simulink model "PV_MPPT_DesktopSim_ST"  (R2018b)
settings: Solver=ode23tb  StartTime=0.0  StopTime=inf  MaxStep=1e-4  RelTol=1e-3
PreLoadFcn:
  | load('EmulatedPV_LowPowerData.mat');
  | 
  | numIrr = 10;
  | ArrayPower = ArrayCurrent.*ArrayVoltage;
InitFcn:
  | Ts = 1e-4;
  | Tc = Ts;
undefined symbols (not defined in the file): ArrayCurrent, ArrayVoltage, DiscIntNeverNeededParam, Irradiance, Tdata
libraries: powerlib x18, simulink x3, powerlib_meascontrol x3
settings Model: Creator=mmishra  LastModifiedBy=jlesage
settings DebuggingCC: LibraryContextMissingDiagnostic=none
settings SFSimCC: SimUseLocalCustomCode=off
settings RTWCC: RTWUseLocalCustomCode=off

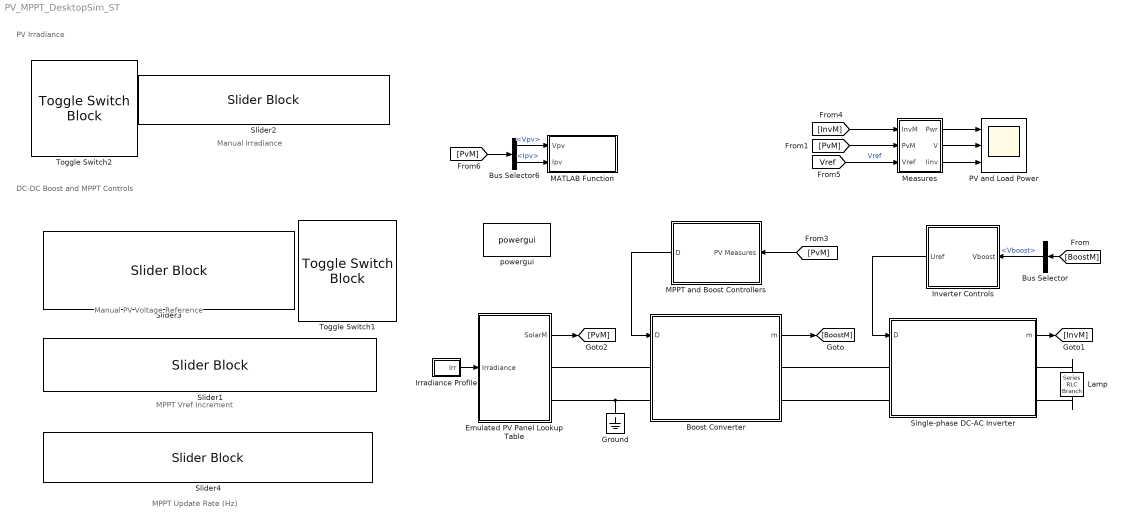
== system PV_MPPT_DesktopSim_ST ==
  note: Manual Irradiance
  note: PV Irradiance
  note: MPPT Update Rate (Hz)
  note: MPPT Vref Increment
  note: DC-DC Boost and MPPT Controls
  note: Manual PV Voltage Reference
  Boost Converter : Subsystem
  Bus Selector : BusSelector  OutputSignals=Vboost
  Bus Selector6 : BusSelector  OutputSignals=Vpv,Ipv
  Emulated PV Panel Lookup Table : Subsystem
      mask Display:
      | image(imread('panel.jpg'))
      | color('yellow')
      | port_label('input',1,'Ir')
      | port_label('output',1,'m')
      | port_label('Rconn',1,'A')
      | port_label('Rconn',2,'B')
  Ground : powerlib/Elements/Ground  LConnTagsString=a
      settings: SourceProductName=Simscape Electrical
  Inverter Controls : Subsystem
  Irradiance Profile : Subsystem
  Lamp : powerlib/Elements/Series RLC Branch  LConnTagsString=__new0  RConnTagsString=__new0  BranchType=R  Resistance=11.5  Inductance=1e-3  SetiL0=off  InitialCurrent=0  Capacitance=1e-6  Setx0=off  InitialVoltage=0  Measurements=None
      settings: SourceProductName=Simscape Electrical
  MATLAB Function : MATLAB Function  TreatAsAtomicUnit=on  SystemSampleTime=1/20
  MPPT and Boost Controllers : Subsystem
  Measures : Subsystem
  PV and Load Power : Scope  NumInputPorts=3
  Single-phase DC-AC Inverter : Subsystem
  Slider1 : SliderBlock  WebBlockId=613  ScaleMax=0.5  TickInterval=0.10000000000000001
  Slider2 : SliderBlock  WebBlockId=612  ScaleMax=0.5  TickInterval=0.10000000000000001
  Slider3 : SliderBlock  WebBlockId=614  ScaleMin=1  ScaleMax=10  TickInterval=1
  Slider4 : SliderBlock  WebBlockId=615  ScaleMin=25  ScaleMax=250  TickInterval=25
  Toggle Switch1 : ToggleSwitchBlock  WebBlockId=610  LabelPosition=Hide
      settings: Values={{'Manual Vref', 'Enable MPPT'}, [0 1]}
  Toggle Switch2 : ToggleSwitchBlock  WebBlockId=611  LabelPosition=Hide
      settings: Values={{'Use Profile', 'Set Irradiance'}, [0 1]}
  powergui : powerlib/powergui  Priority=1  SimulationMode=Discrete  SampleTime=Ts  frequency=60  Iterations=50  frequencyindice=0  Pbase=100e6  ErrMax=1e-4  UnitsV=kV  UnitsW=MW  buscounter=0  FunctionMessages=off  echomessages=off  EnableUseOfTLC=off  CurrentSourceSwitches=off  DisableSnubberDevices=off  DisableRonSwitches=off  DisableVfSwitches=off  DisplayEquations=off  SolverType=Tustin/Backward Euler (TBE)  Interpol=off  ExternalGateDelay=off  methode=off  Ts=100  x0status=blocks  SPID=on  SwTol=0  HookPort=off  RestoreLinks=warning  ResistiveCurrentMeasurement=off  Frange=[0:2:500]  Ylog=off  Xlog=on  ShowGrid=off  save=off  variable=ZData  structure=0  ZoomFFT=off  StartTime=0.0  cycles=1  DisplayStyle=1  fundamental=60  FreqAxis=off  MaxFrequency=1000  frequencyindicesteady=1  RmsSteady=1  display=off
      settings: SourceProductName=Simscape Electrical
  wires:
  Irradiance Profile/1(Irr) -> Emulated PV Panel Lookup Table/1(Irradiance)
  Single-phase DC-AC Inverter/1(m) -> [InvM]
  Emulated PV Panel Lookup Table/1(SolarM) -> [PvM]
  MPPT and Boost Controllers/1(D) -> Boost Converter/1(D)
  Boost Converter/1(m) -> [BoostM]
  [PvM] -> MPPT and Boost Controllers/1(PV Measures)
  Bus Selector/1 -> Inverter Controls/1(Vboost)  "<Vboost>"
  Inverter Controls/1(Uref) -> Single-phase DC-AC Inverter/1(D)
  [BoostM] -> Bus Selector/1
  Bus Selector6/1 -> MATLAB Function/1(Vpv)  "<Vpv>"
  Bus Selector6/2 -> MATLAB Function/2(Ipv)  "<Ipv>"
  [PvM] -> Bus Selector6/1
  [InvM] -> Measures/1(InvM)
  [PvM] -> Measures/2(PvM)
  [Vref] -> Measures/3(Vref)  "Vref"
  Measures/1(Pwr) -> PV and Load Power/1
  Measures/2(V) -> PV and Load Power/2
  Measures/3(Iinv) -> PV and Load Power/3
  connections:
  Ground/LConn1 -- Emulated PV Panel Lookup Table/RConn2 -- Boost Converter/LConn2
  Emulated PV Panel Lookup Table/RConn1 -- Boost Converter/LConn1
  Lamp/RConn1 -- Single-phase DC-AC Inverter/RConn2
  Single-phase DC-AC Inverter/LConn1 -- Boost Converter/RConn1
  Single-phase DC-AC Inverter/LConn2 -- Boost Converter/RConn2
  Lamp/LConn1 -- Single-phase DC-AC Inverter/RConn1

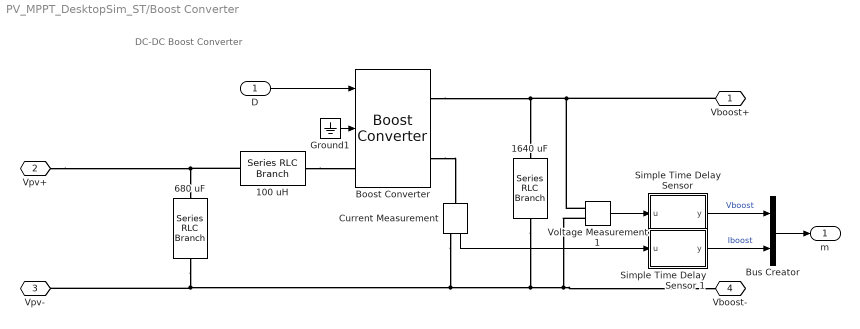
== system PV_MPPT_DesktopSim_ST/Boost Converter ==
  note: DC-DC Boost Converter
  D : Inport
  100 uH : powerlib/Elements/Series RLC Branch  LConnTagsString=__new0  RConnTagsString=__new0  BranchType=L  Resistance=1  Inductance=100e-6  SetiL0=off  InitialCurrent=0  Capacitance=1e-6  Setx0=off  InitialVoltage=0  Measurements=None
      settings: SourceProductName=Simscape Electrical
  1640 uF : powerlib/Elements/Series RLC Branch  LConnTagsString=__new0  RConnTagsString=__new0  BranchType=C  Resistance=1  Inductance=1e-3  SetiL0=off  InitialCurrent=0  Capacitance=1640e-6  Setx0=off  InitialVoltage=30  Measurements=None
      settings: SourceProductName=Simscape Electrical
  680 uF : powerlib/Elements/Series RLC Branch  LConnTagsString=__new0  RConnTagsString=__new0  BranchType=C  Resistance=1e-3  Inductance=1e-3  SetiL0=off  InitialCurrent=0  Capacitance=680e-6  Setx0=off  InitialVoltage=20  Measurements=None
      settings: SourceProductName=Simscape Electrical
  "Boost Converter " : powerlib/Power Electronics/Boost Converter  ModelType=Average model (D-controlled)  Ron=1e-3  Rs=1e6  Cs=inf  Vforward=[0,0.8]  Ron_Diode=1e-3  Rs_Diode=1e6  Cs_Diode=inf  Vf_Diode=0.8  Rs_CurrentSource=inf
      settings: SourceProductName=Simscape Electrical  SourceProductBaseCode=PS
  Bus Creator : BusCreator  Inputs=2
  Current Measurement : powerlib/Measurements/Current Measurement  PhasorSimulation=off  OutputType=Complex  PSBequivalent=0
      settings: SourceProductName=Simscape Electrical
  Ground1 : Ground
  "Simple Time Delay Sensor " : Subsystem  mask{Ts=Ts, Tau=0.0001}
      mask prompts: Ts "Sample Time, [s]"; Tau "Time Constant, Tau [s]"
      mask help: Simple Sensor
      mask Display: fprintf('1\n------------\n(1 + s Tau)');
  Simple Time Delay Sensor 1 : Subsystem  mask{Ts=Ts, Tau=0.0001}
      mask prompts: Ts "Sample Time, [s]"; Tau "Time Constant, Tau [s]"
      mask help: Simple Sensor
      mask Display: fprintf('1\n------------\n(1 + s Tau)');
  Voltage Measurement1 : powerlib/Measurements/Voltage Measurement  PhasorSimulation=off  OutputType=Complex  PSBequivalent=0
      settings: SourceProductName=Simscape Electrical
  Vboost+ : PMIOPort  Side=Right
  Vpv+ : PMIOPort  Port=2  Side=Left
  Vpv- : PMIOPort  Port=3  Side=Left
  Vboost- : PMIOPort  Port=4  Side=Right
  m : Outport
  wires:
  Ground1/1 -> "Boost Converter "/2
  Current Measurement/1 -> Simple Time Delay Sensor 1/1(u)
  Voltage Measurement1/1 -> "Simple Time Delay Sensor "/1(u)
  Bus Creator/1 -> m/1
  "Simple Time Delay Sensor "/1(y) -> Bus Creator/1  "Vboost"
  Simple Time Delay Sensor 1/1(y) -> Bus Creator/2  "Iboost"
  D/1 -> "Boost Converter "/1
  connections:
  100 uH/LConn1 -- Vpv+/RConn1 -- 680 uF/LConn1
  "Boost Converter "/RConn2 -- Current Measurement/LConn1
  100 uH/RConn1 -- "Boost Converter "/LConn1
  Voltage Measurement1/LConn1 -- Vboost+/RConn1 -- "Boost Converter "/RConn1 -- 1640 uF/LConn1
  680 uF/RConn1 -- Vboost-/RConn1 -- Voltage Measurement1/LConn2 -- 1640 uF/RConn1 -- Current Measurement/RConn1 -- Vpv-/RConn1

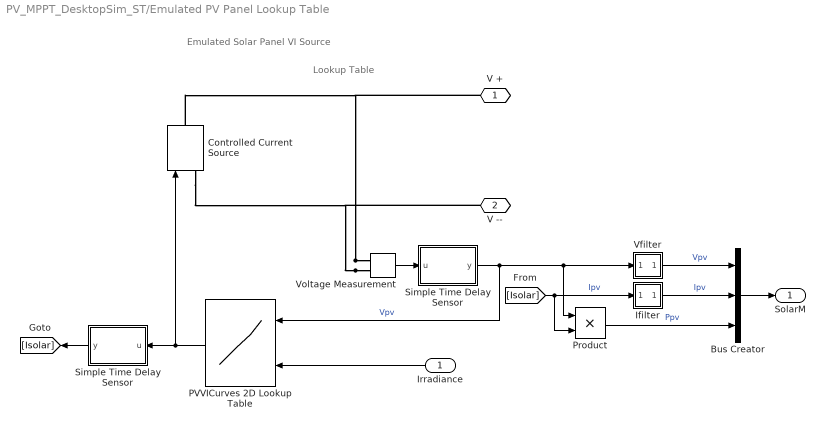
== system PV_MPPT_DesktopSim_ST/Emulated PV Panel Lookup Table ==
  note: Lookup Table
  note: Emulated Solar Panel VI Source
  Irradiance : Inport
  Bus Creator : BusCreator  Inputs=3
  Controlled Current Source : powerlib/Electrical Sources/Controlled Current Source  Initialize=on  Source_Type=AC  Amplitude=0  Phase=0  Frequency=0  Measurements=None
      settings: SourceProductName=Simscape Electrical
  Ifilter : Subsystem  mask{Tf=0.01}
      mask prompts: Tf "Filter Time Constant"
  PVVICurves 2D Lookup Table : Lookup_n-D  BreakpointsForDimension1=ArrayVoltage  BreakpointsForDimension2=Irradiance  Table=ArrayCurrent  InternalRulePriority=Speed  RndMeth=Simplest  InputSameDT=on
  Product : Product
  Simple Time Delay Sensor : Subsystem  mask{Ts=Ts, Tau=0.0001}
      mask prompts: Ts "Sample Time, [s]"; Tau "Time Constant, Tau [s]"
      mask help: Simple Sensor
      mask Display: fprintf('1\n------------\n(1 + s Tau)');
  "Simple Time Delay Sensor " : Subsystem  mask{Ts=Ts, Tau=0.0001}
      mask prompts: Ts "Sample Time, [s]"; Tau "Time Constant, Tau [s]"
      mask help: Simple Sensor
      mask Display: fprintf('1\n------------\n(1 + s Tau)');
  Vfilter : Subsystem  mask{Tf=0.01}
      mask prompts: Tf "Filter Time Constant"
  Voltage Measurement : powerlib/Measurements/Voltage Measurement  PhasorSimulation=off  OutputType=Complex  PSBequivalent=0
      settings: SourceProductName=Simscape Electrical
  V + : PMIOPort  Side=Right
  V -- : PMIOPort  Port=2  Side=Right
  SolarM : Outport
  wires:
  Irradiance/1 -> PVVICurves 2D Lookup Table/2
  PVVICurves 2D Lookup Table/1 -> Simple Time Delay Sensor/1(u), Controlled Current Source/1
  Bus Creator/1 -> SolarM/1
  [Isolar] -> Product/2, Ifilter/1(u)  "Ipv"
  Product/1 -> Bus Creator/3  "Ppv"
  Simple Time Delay Sensor/1(y) -> [Isolar]
  "Simple Time Delay Sensor "/1(y) -> Product/1, Vfilter/1(u), PVVICurves 2D Lookup Table/1  "Vpv"
  Voltage Measurement/1 -> "Simple Time Delay Sensor "/1(u)
  Vfilter/1(y) -> Bus Creator/1  "Vpv"
  Ifilter/1(y) -> Bus Creator/2  "Ipv"
  connections:
  Voltage Measurement/LConn2 -- Controlled Current Source/LConn1 -- V --/RConn1
  Voltage Measurement/LConn1 -- Controlled Current Source/RConn1 -- V +/RConn1

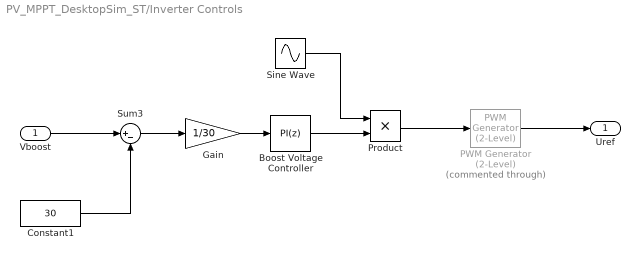
== system PV_MPPT_DesktopSim_ST/Inverter Controls ==
  Vboost : Inport
  Boost Voltage Controller : simulink/Continuous/PID Controller  Controller=PI  Form=Parallel  TimeDomain=Discrete-time  SampleTime=Tc  IntegratorMethod=Forward Euler  FilterMethod=Forward Euler  ControllerParametersSource=internal  P=3  I=250  D=0  UseFilter=on  N=100  TunerSelectOption=Transfer Function Based (PID Tuner App)  InitialConditionSource=internal  InitialConditionForIntegrator=1  InitialConditionForFilter=0  DifferentiatorICPrevScaledInput=0  ExternalReset=none  TrackingMode=off  Kt=1  LimitOutput=on  UpperSaturationLimit=1  LowerSaturationLimit=0  LinearizeAsGain=on  AntiWindupMode=clamping  Kb=1  POutMin=[]  POutMax=[]  IOutMin=[]  IOutMax=[]  DOutMin=[]  DOutMax=[]  NOutMin=[]  NOutMax=[]  SumOutMin=[]  SumOutMax=[]  SaturationOutMin=[]  SaturationOutMax=[]  PParamMin=[]  PParamMax=[]  IParamMin=[]  IParamMax=[]  DParamMin=[]  DParamMax=[]  NParamMin=[]  NParamMax=[]  KbParamMin=[]  KbParamMax=[]  KtParamMin=[]  KtParamMax=[]  KbOutMin=[]  KbOutMax=[]  KtOutMin=[]  KtOutMax=[]  IntegratorOutMin=[]  IntegratorOutMax=[]  FilterOutMin=[]  FilterOutMax=[]  SumI1OutMin=[]  SumI1OutMax=[]  SumI2OutMin=[]  SumI2OutMax=[]  SumI3OutMin=[]  SumI3OutMax=[]  SumI4OutMin=[]  SumI4OutMax=[]  SumDOutMin=[]  SumDOutMax=[]  DifferentiatorOutMin=[]  DifferentiatorOutMax=[]  FilterDiffOutCoefMin=[]  FilterDiffOutCoefMax=[]  ReciprocalOutMin=[]  ReciprocalOutMax=[]  SumDenOutMin=[]  SumDenOutMax=[]  SumNumOutMin=[]  SumNumOutMax=[]  DivideOutMin=[]  DivideOutMax=[]  IntegratorContinuousStateAttributes=''  IntegratorStateMustResolveToSignalObject=off  IntegratorRTWStateStorageClass=Auto  FilterContinuousStateAttributes=''  FilterStateMustResolveToSignalObject=off  FilterRTWStateStorageClass=Auto  ParallelPVariant=InternalParameters  IdealPVariant=Disabled  IVariant=InternalParameters  DVariant=Disabled  IntegratorVariant=Discrete  SatVariant=Enabled  AWVariant=DiscClampingParallel  PCopyVariant=Disabled  TRVariant=Disabled  FdbkBlocksVariant=Forward  IdealPFdbkVariant=Disabled  SatFdbkVariant=Disabled  DerivativeFilterVariant=Disabled  NVariant=Disabled  NCopyVariant=Disabled_SignalSpec  FilterICVariant=Disabled  IntegratorICVariant=InternalICs  ExternalResetVariant=Disabled  TRSumVariant=Passthrough  SumFdbkVariant=Disabled  SumVariant=Sum_PI
  Constant1 : Constant  Value=30
  Gain : Gain  Gain=1/30
  "PWM Generator (2-Level) " : powerlib_meascontrol/Pulse & Signal Generators/PWM Generator (2-Level)  Commented=through  ModulatorType=Single-phase full-bridge (4 pulses)  ModulatorMode=Unsynchronized  Fc=6000  Pc=90  nF=27  MinMax="[ -1  1 ]"  SamplingTechnique=Natural  ModulatingSignals=off  m=0.8  Freq=60  Phase=0  Ts=Ts  ShowCarrierOutport=off
  Product : Product
  Sine Wave : Sin  Frequency=2*pi*60  SampleTime=Tc
  Sum3 : Sum  Inputs=|+-
  Uref : Outport
  wires:
  Constant1/1 -> Sum3/2
  Sine Wave/1 -> Product/1
  Boost Voltage Controller/1 -> Product/2
  Sum3/1 -> Gain/1
  Vboost/1 -> Sum3/1
  Gain/1 -> Boost Voltage Controller/1
  Product/1 -> "PWM Generator (2-Level) "/1
  "PWM Generator (2-Level) "/1 -> Uref/1

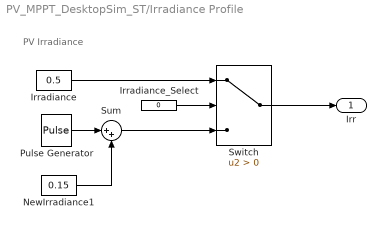
== system PV_MPPT_DesktopSim_ST/Irradiance Profile ==
  note: PV Irradiance
  Irradiance : Constant  Value=0.5  OutDataTypeStr=single
  Irradiance_Select : Constant  Value=0  OutDataTypeStr=single
  NewIrradiance1 : Constant  Value=0.15  OutDataTypeStr=single
  Pulse Generator : DiscretePulseGenerator  PulseType=Time based  Amplitude=0.15  Period=10  PulseWidth=50
  Sum : Sum  Inputs=|++
  Switch : Switch  Criteria=u2 > Threshold
  Irr : Outport
  wires:
  NewIrradiance1/1 -> Sum/2
  Pulse Generator/1 -> Sum/1
  Sum/1 -> Switch/3
  Irradiance/1 -> Switch/1
  Switch/1 -> Irr/1
  Irradiance_Select/1 -> Switch/2

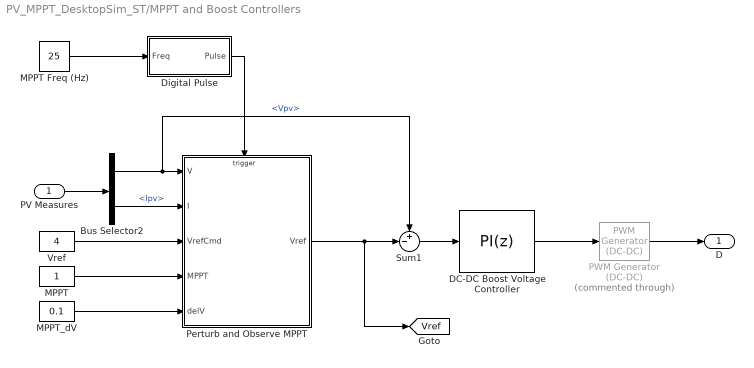
== system PV_MPPT_DesktopSim_ST/MPPT and Boost Controllers ==
  PV Measures : Inport
  Bus Selector2 : BusSelector  OutputSignals=Vpv,Ipv
  DC-DC Boost Voltage Controller : simulink/Continuous/PID Controller  Controller=PI  Form=Parallel  TimeDomain=Discrete-time  SampleTime=Tc  IntegratorMethod=Forward Euler  FilterMethod=Forward Euler  ControllerParametersSource=internal  P=0.015  I=2.5  D=0  UseFilter=on  N=100  TunerSelectOption=Transfer Function Based (PID Tuner App)  InitialConditionSource=internal  InitialConditionForIntegrator=0  InitialConditionForFilter=0  DifferentiatorICPrevScaledInput=0  ExternalReset=none  TrackingMode=off  Kt=1  LimitOutput=off  UpperSaturationLimit=0.9  LowerSaturationLimit=0  LinearizeAsGain=on  AntiWindupMode=clamping  Kb=1  POutMin=[]  POutMax=[]  IOutMin=[]  IOutMax=[]  DOutMin=[]  DOutMax=[]  NOutMin=[]  NOutMax=[]  SumOutMin=[]  SumOutMax=[]  SaturationOutMin=[]  SaturationOutMax=[]  PParamMin=[]  PParamMax=[]  IParamMin=[]  IParamMax=[]  DParamMin=[]  DParamMax=[]  NParamMin=[]  NParamMax=[]  KbParamMin=[]  KbParamMax=[]  KtParamMin=[]  KtParamMax=[]  KbOutMin=[]  KbOutMax=[]  KtOutMin=[]  KtOutMax=[]  IntegratorOutMin=[]  IntegratorOutMax=[]  FilterOutMin=[]  FilterOutMax=[]  SumI1OutMin=[]  SumI1OutMax=[]  SumI2OutMin=[]  SumI2OutMax=[]  SumI3OutMin=[]  SumI3OutMax=[]  SumI4OutMin=[]  SumI4OutMax=[]  SumDOutMin=[]  SumDOutMax=[]  DifferentiatorOutMin=[]  DifferentiatorOutMax=[]  FilterDiffOutCoefMin=[]  FilterDiffOutCoefMax=[]  ReciprocalOutMin=[]  ReciprocalOutMax=[]  SumDenOutMin=[]  SumDenOutMax=[]  SumNumOutMin=[]  SumNumOutMax=[]  DivideOutMin=[]  DivideOutMax=[]  IntegratorContinuousStateAttributes=''  IntegratorStateMustResolveToSignalObject=off  IntegratorRTWStateStorageClass=Auto  FilterContinuousStateAttributes=''  FilterStateMustResolveToSignalObject=off  FilterRTWStateStorageClass=Auto  ParallelPVariant=InternalParameters  IdealPVariant=Disabled  IVariant=InternalParameters  DVariant=Disabled  IntegratorVariant=Discrete  SatVariant=Disabled  AWVariant=Passthrough  PCopyVariant=Disabled  TRVariant=Disabled  FdbkBlocksVariant=Forward  IdealPFdbkVariant=Disabled  SatFdbkVariant=Disabled  DerivativeFilterVariant=Disabled  NVariant=Disabled  NCopyVariant=Disabled_SignalSpec  FilterICVariant=Disabled  IntegratorICVariant=InternalICs  ExternalResetVariant=Disabled  TRSumVariant=Passthrough  SumFdbkVariant=Disabled  SumVariant=Sum_PI
  Digital Pulse : Subsystem  mask{Ts=Tc, Duty=0.5}
      mask prompts: Ts "Sample Rate [s]"; Duty "Duty Cycle [0-1]"
  MPPT : Constant
  MPPT Freq (Hz) : Constant  Value=25
  MPPT_dV : Constant  Value=0.1
  PWM Generator (DC-DC) : powerlib_meascontrol/Pulse & Signal Generators/PWM Generator (DC-DC)  Commented=through  Fsw=5000  Ts=Ts
      settings: SourceProductName=Simscape Electrical
  Perturb and Observe MPPT : Stateflow chart  TreatAsAtomicUnit=on  SystemSampleTime=Tdata
  Sum1 : Sum  Inputs=+-|
  Vref : Constant  Value=4
  D : Outport
  tag scope: Vref=global
  wires:
  PV Measures/1 -> Bus Selector2/1
  Digital Pulse/1(Pulse) -> Perturb and Observe MPPT/Trigger
  MPPT Freq (Hz)/1 -> Digital Pulse/1(Freq)
  MPPT_dV/1 -> Perturb and Observe MPPT/5(delV)
  Vref/1 -> Perturb and Observe MPPT/3(VrefCmd)
  Sum1/1 -> DC-DC Boost Voltage Controller/1
  MPPT/1 -> Perturb and Observe MPPT/4(MPPT)
  Bus Selector2/1 -> Perturb and Observe MPPT/1(V), Sum1/1  "<Vpv>"
  Perturb and Observe MPPT/1(Vref) -> [Vref], Sum1/2
  Bus Selector2/2 -> Perturb and Observe MPPT/2(I)  "<Ipv>"
  DC-DC Boost Voltage Controller/1 -> PWM Generator (DC-DC)/1
  PWM Generator (DC-DC)/1 -> D/1

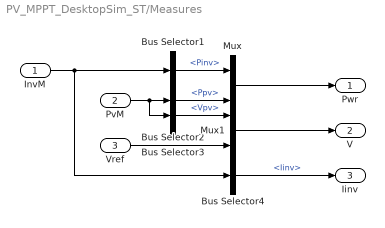
== system PV_MPPT_DesktopSim_ST/Measures ==
  InvM : Inport
  PvM : Inport  Port=2
  Vref : Inport  Port=3
  Bus Selector1 : BusSelector  OutputSignals=Pinv
  Bus Selector2 : BusSelector  OutputSignals=Ppv
  Bus Selector3 : BusSelector  OutputSignals=Vpv
  Bus Selector4 : BusSelector  OutputSignals=Iinv
  Mux : Mux  Inputs=2
  Mux1 : Mux  Inputs=2
  Pwr : Outport
  V : Outport  Port=2
  Iinv : Outport  Port=3
  wires:
  Bus Selector2/1 -> Mux/2  "<Ppv>"
  PvM/1 -> Bus Selector3/1, Bus Selector2/1
  Mux/1 -> Pwr/1
  Bus Selector1/1 -> Mux/1  "<Pinv>"
  Bus Selector3/1 -> Mux1/1  "<Vpv>"
  Bus Selector4/1 -> Iinv/1  "<Iinv>"
  Mux1/1 -> V/1
  Vref/1 -> Mux1/2
  InvM/1 -> Bus Selector4/1, Bus Selector1/1

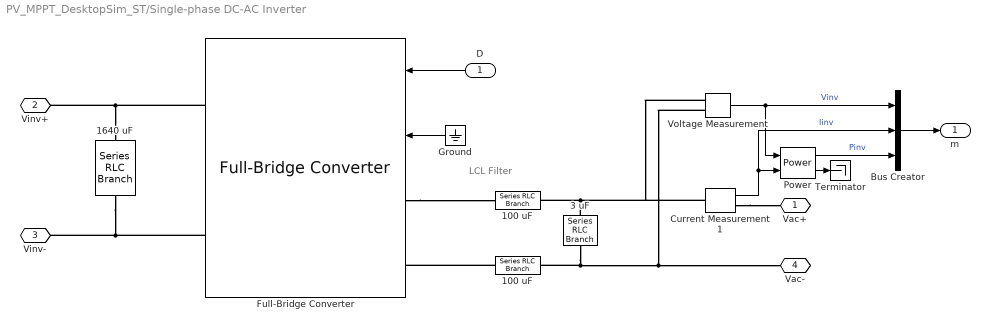
== system PV_MPPT_DesktopSim_ST/Single-phase DC-AC Inverter ==
  note: LCL Filter
  D : Inport
  100 uF : powerlib/Elements/Series RLC Branch  LConnTagsString=__new0  RConnTagsString=__new0  BranchType=L  Resistance=1  Inductance=100e-6  SetiL0=off  InitialCurrent=0  Capacitance=1e-6  Setx0=off  InitialVoltage=0  Measurements=None
      settings: SourceProductName=Simscape Electrical
  "100 uF " : powerlib/Elements/Series RLC Branch  LConnTagsString=__new0  RConnTagsString=__new0  BranchType=L  Resistance=1  Inductance=100e-6  SetiL0=off  InitialCurrent=0  Capacitance=1e-6  Setx0=off  InitialVoltage=0  Measurements=None
      settings: SourceProductName=Simscape Electrical
  "1640 uF " : powerlib/Elements/Series RLC Branch  LConnTagsString=__new0  RConnTagsString=__new0  BranchType=RC  Resistance=0.05  Inductance=1e-3  SetiL0=off  InitialCurrent=0  Capacitance=1640e-6  Setx0=off  InitialVoltage=0  Measurements=None
      settings: SourceProductName=Simscape Electrical
  3 uF : powerlib/Elements/Series RLC Branch  LConnTagsString=__new0  RConnTagsString=__new0  BranchType=C  Resistance=1  Inductance=1e-3  SetiL0=off  InitialCurrent=0  Capacitance=3e-6  Setx0=off  InitialVoltage=0  Measurements=None
      settings: SourceProductName=Simscape Electrical
  Bus Creator : BusCreator  Inputs=3
  Current Measurement1 : powerlib/Measurements/Current Measurement  PhasorSimulation=off  OutputType=Complex  PSBequivalent=0
      settings: SourceProductName=Simscape Electrical
  Full-Bridge Converter : powerlib/Power Electronics/Full-Bridge Converter  ModelType=Average model (Uref-controlled)  Ron=1e-3  Rs=1e6  Cs=inf  Vforward=[0,0]  Ron_Diode=1e-3  Rs_Diode=1e6  Cs_Diode=inf  Vf_Diode=1e-3  Rs_CurrentSource=inf
      settings: SourceProductName=Simscape Electrical  SourceProductBaseCode=PS
  Ground : Ground
  Power : powerlib_meascontrol/Measurements/Power  Freq=60  Vinit=[1, 0]  Iinit=[1, 0]  Ts=Ts
      settings: SourceProductName=Simscape Electrical
  Terminator : Terminator
  Voltage Measurement : powerlib/Measurements/Voltage Measurement  PhasorSimulation=off  OutputType=Complex  PSBequivalent=0
      settings: SourceProductName=Simscape Electrical
  Vac+ : PMIOPort  Side=Right
  Vinv+ : PMIOPort  Port=2  Side=Left
  Vinv- : PMIOPort  Port=3  Side=Left
  Vac- : PMIOPort  Port=4  Side=Right
  m : Outport
  wires:
  Ground/1 -> Full-Bridge Converter/2
  D/1 -> Full-Bridge Converter/1
  Bus Creator/1 -> m/1
  Power/1 -> Bus Creator/3  "Pinv"
  Voltage Measurement/1 -> Bus Creator/1, Power/1  "Vinv"
  Current Measurement1/1 -> Power/2, Bus Creator/2  "Iinv"
  Power/2 -> Terminator/1
  connections:
  Full-Bridge Converter/RConn1 -- "1640 uF "/LConn1 -- Vinv+/RConn1
  3 uF/RConn1 -- Vac-/RConn1 -- Voltage Measurement/LConn2 -- "100 uF "/RConn1
  "1640 uF "/RConn1 -- Full-Bridge Converter/RConn2 -- Vinv-/RConn1
  "100 uF "/LConn1 -- Full-Bridge Converter/LConn2
  Full-Bridge Converter/LConn1 -- 100 uF/LConn1
  3 uF/LConn1 -- Current Measurement1/LConn1 -- Voltage Measurement/LConn1 -- 100 uF/RConn1
  Current Measurement1/RConn1 -- Vac+/RConn1

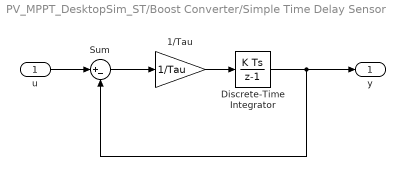
== system PV_MPPT_DesktopSim_ST/Boost Converter/Simple Time Delay Sensor  ==
  u : Inport
  1/Tau : Gain  Gain=1/Tau
  Discrete-Time Integrator : DiscreteIntegrator  SampleTime=Ts  ICPrevOutput=DiscIntNeverNeededParam  ICPrevScaledInput=DiscIntNeverNeededParam
  Sum : Sum  Inputs=|+-
  y : Outport
  wires:
  Discrete-Time Integrator/1 -> Sum/2, y/1
  u/1 -> Sum/1
  Sum/1 -> 1/Tau/1
  1/Tau/1 -> Discrete-Time Integrator/1

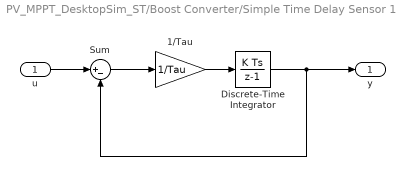
== system PV_MPPT_DesktopSim_ST/Boost Converter/Simple Time Delay Sensor 1 ==
  u : Inport
  1/Tau : Gain  Gain=1/Tau
  Discrete-Time Integrator : DiscreteIntegrator  SampleTime=Ts  ICPrevOutput=DiscIntNeverNeededParam  ICPrevScaledInput=DiscIntNeverNeededParam
  Sum : Sum  Inputs=|+-
  y : Outport
  wires:
  1/Tau/1 -> Discrete-Time Integrator/1
  Sum/1 -> 1/Tau/1
  u/1 -> Sum/1
  Discrete-Time Integrator/1 -> y/1, Sum/2

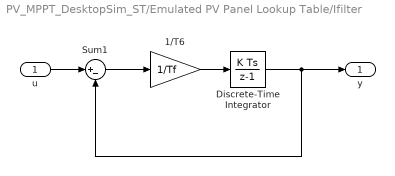
== system PV_MPPT_DesktopSim_ST/Emulated PV Panel Lookup Table/Ifilter ==
  u : Inport
  1/T6 : Gain  Gain=1/Tf
  Discrete-Time Integrator : DiscreteIntegrator  SampleTime=Tc  ICPrevOutput=DiscIntNeverNeededParam  ICPrevScaledInput=DiscIntNeverNeededParam
  Sum1 : Sum  Inputs=|+-
  y : Outport
  wires:
  Sum1/1 -> 1/T6/1
  Discrete-Time Integrator/1 -> Sum1/2, y/1
  u/1 -> Sum1/1
  1/T6/1 -> Discrete-Time Integrator/1

== system PV_MPPT_DesktopSim_ST/Emulated PV Panel Lookup Table/Simple Time Delay Sensor ==
  u : Inport
  1/Tau : Gain  Gain=1/Tau
  Discrete-Time Integrator : DiscreteIntegrator  SampleTime=Ts  ICPrevOutput=DiscIntNeverNeededParam  ICPrevScaledInput=DiscIntNeverNeededParam
  Sum : Sum  Inputs=|+-
  y : Outport
  wires:
  1/Tau/1 -> Discrete-Time Integrator/1
  Sum/1 -> 1/Tau/1
  u/1 -> Sum/1
  Discrete-Time Integrator/1 -> y/1, Sum/2

== system PV_MPPT_DesktopSim_ST/Emulated PV Panel Lookup Table/Simple Time Delay Sensor  ==
  u : Inport
  1/Tau : Gain  Gain=1/Tau
  Discrete-Time Integrator : DiscreteIntegrator  SampleTime=Ts  ICPrevOutput=DiscIntNeverNeededParam  ICPrevScaledInput=DiscIntNeverNeededParam
  Sum : Sum  Inputs=|+-
  y : Outport
  wires:
  Discrete-Time Integrator/1 -> Sum/2, y/1
  u/1 -> Sum/1
  Sum/1 -> 1/Tau/1
  1/Tau/1 -> Discrete-Time Integrator/1

== system PV_MPPT_DesktopSim_ST/Emulated PV Panel Lookup Table/Vfilter ==
  u : Inport
  1/T6 : Gain  Gain=1/Tf
  Discrete-Time Integrator : DiscreteIntegrator  SampleTime=Tc  ICPrevOutput=DiscIntNeverNeededParam  ICPrevScaledInput=DiscIntNeverNeededParam
  Sum1 : Sum  Inputs=|+-
  y : Outport
  wires:
  1/T6/1 -> Discrete-Time Integrator/1
  u/1 -> Sum1/1
  Discrete-Time Integrator/1 -> y/1, Sum1/2
  Sum1/1 -> 1/T6/1

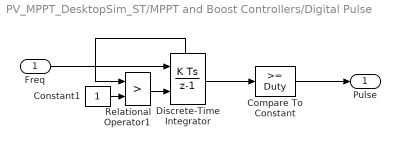
== system PV_MPPT_DesktopSim_ST/MPPT and Boost Controllers/Digital Pulse ==
  Freq : Inport
  Compare To Constant : simulink/Logic and Bit Operations/Compare To Constant  relop=>=  const=Duty  OutDataTypeStr=boolean
  Constant1 : Constant
  Discrete-Time Integrator : DiscreteIntegrator  ExternalReset=rising  SampleTime=Ts  ShowStatePort=on  ICPrevOutput=DiscIntNeverNeededParam  ICPrevScaledInput=DiscIntNeverNeededParam
  Relational Operator1 : RelationalOperator  Operator=>  OutDataTypeStr=boolean  RndMeth=Nearest
  Pulse : Outport
  wires:
  Relational Operator1/1 -> Discrete-Time Integrator/2
  Constant1/1 -> Relational Operator1/2
  Compare To Constant/1 -> Pulse/1
  Discrete-Time Integrator/State -> Relational Operator1/1
  Discrete-Time Integrator/1 -> Compare To Constant/1
  Freq/1 -> Discrete-Time Integrator/1

== matlab function PV_MPPT_DesktopSim_ST/MATLAB Function ==
  settings: updateMethod=DISCRETE
  data: Vpv input; Ipv input; ArrayPower parameter; ArrayVoltage parameter; numIrr parameter
function plotPower(Vpv,Ipv, ArrayPower,ArrayVoltage, numIrr)

    persistent irrPlot powerPlot
%     coder.extrinsic('legend');    
    
    if isempty(irrPlot)
        
        idx = 1:find(ArrayPower(:,numIrr) > 0,1,'last')+2;
                        
        figure(1);
        irrPlot = plot(ArrayVoltage(idx),ArrayPower(idx,1:numIrr)); hold on;
        grid on;
        
        xlabel('PV Voltage [V]');
        ylabel('PV Power [W]');
        title('PV Power Output');
        
        powerPlot = plot(Vpv,Vpv*Ipv,'ro'); 
%         legend('50 W/m^2','100 W/m^2','150 W/m^2','200 W/m^2','250 W/m^2','300 W/m^2',...
%             '350 W/m^2','400 W/m^2','450 W/m^2','500 W/m^2','PV Power');
        hold off;
        
    else 
        set(powerPlot,'XData',Vpv,'YData',Vpv*Ipv);
    end
    
end

== stateflow chart PV_MPPT_DesktopSim_ST/MPPT and Boost Controllers/Perturb and Observe MPPT ==
  state DisableMPPT
    during:
    Vref = VrefCmd;
    Vref_prev = VrefCmd;
  state EnableMPPT
    state Compute_Power
      entry:
      P = V*I;
    state Calculate_Difference
      entry:
      deltaP = P - Pprev;
      deltaV = V - Vprev;
    state Decrement_Vref
      entry:
      Vref = Vref_prev - delV;
    state Increment_Vref
      entry:
      Vref = Vref_prev + delV;
    state Save_PreviousValues
      entry:
      Pprev = P; Vprev = V;
    state Clamp_VrefMax
      entry:
      Vref = VrefMax;
    state Clamp_VrefMin
      entry:
      Vref = VrefMin;
    (default) -> Compute_Power
    (junction 76) -> Compute_Power
    (junction 53) -> (junction 76) : {Vref_prev = Vref;}
    Compute_Power -> Calculate_Difference
    Calculate_Difference -> (junction 13) [order 1] : [deltaP < 0]
    Calculate_Difference -> (junction 14) [order 2] : [deltaP >= 0]
    (junction 13) -> Increment_Vref [order 2] : [deltaV < 0]
    (junction 14) -> Decrement_Vref [order 1] : [deltaV <= 0]
    (junction 13) -> Decrement_Vref [order 1] : [deltaV >= 0]
    (junction 14) -> Increment_Vref [order 2] : [deltaV > 0]
    Decrement_Vref -> Save_PreviousValues
    Increment_Vref -> Save_PreviousValues
    Save_PreviousValues -> (junction 53) [order 3]
    (junction 73) -> (junction 53)
    Save_PreviousValues -> Clamp_VrefMax [order 1] : [Vref >= VrefMax]
    Save_PreviousValues -> Clamp_VrefMin [order 2] : [Vref <= VrefMin]
    Clamp_VrefMax -> (junction 70)
    Clamp_VrefMin -> (junction 50)
    (junction 70) -> (junction 50)
    (junction 50) -> (junction 73)
  (default) -> DisableMPPT
  (junction 91) -> DisableMPPT
  EnableMPPT -> (junction 91) : [MPPT ~= 1]
  DisableMPPT -> EnableMPPT : [MPPT == 1]
  data: P local double =0; k local double =0; Psum local double =0; Vsum local double =0; Vavg local double =0; Pavg local double =0; deltaP local double =0; Pprev local double =0; Vprev local double =0; deltaV local double =0; Vref output double =5; Vref_prev local double =5; VrefMax constant double =28; VrefMin constant double =1; V input double; I input double; VrefCmd input double; MPPT input double; delV input double
  events: event input RISING_EDGE_EVENT
